simulink model "Task_f"  (R2025b)
settings: Solver=VariableStepAuto  StartTime=0.0  StopTime=10000  RelTol=1e-3
model workspace (MAT data in the model file):
  F = [0.06  0  0; 0  0.06  0; 0  0  0]
values from neighbouring files (symbols this model uses):
  A = [ -(1/(R1*C1) + 1/(R2*C1)),   1/(R2*C1),                 0 ... (first row only)    [Lab_Prep.m]    (also in Lab_Session.m = [ -(k1 + k12),      k12,            0)
  b = [1/(R1*C1); 0; 0]    [Lab_Prep.m]    (also in Lab_Session.m = [kin; 0; 0])
  C = [0, 0, 1]    [Lab_Prep.m]    (also in Lab_Session.m = [0 0 1])
  D = [0 0]    [Lab_Session.m]
settings Model: Creator=DemoBox  LastModifiedBy=DemoBox

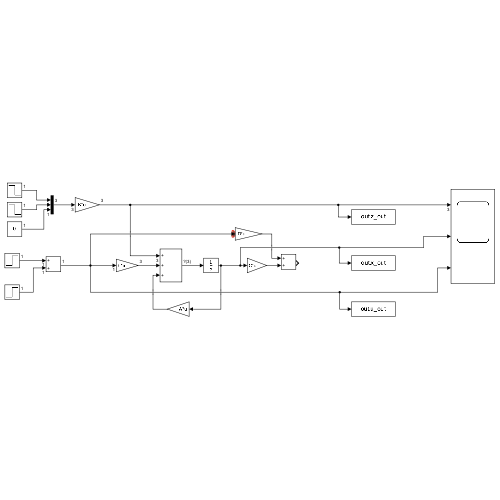
[thumbnail: Simulink's stored preview of the top-level diagram]
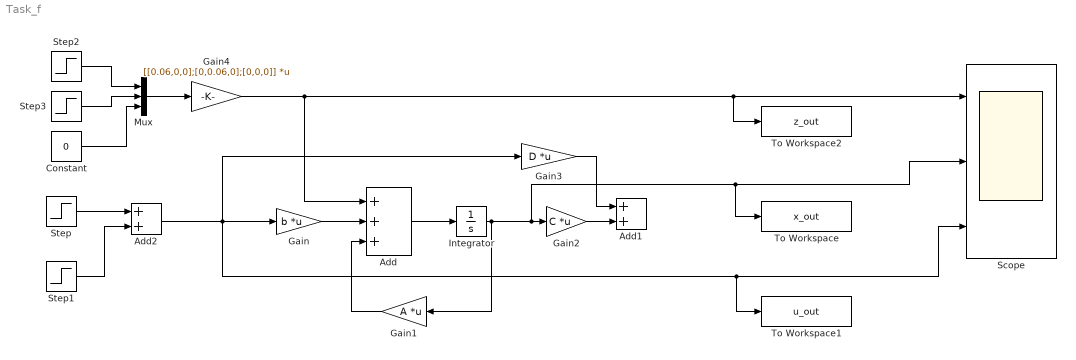
== system Task_f ==
  Add : Sum  Inputs=+++
  Add1 : Sum
  Add2 : Sum
  Constant : Constant  Value=0
  Gain : Gain  Gain=b  Multiplication=Matrix(K*u)
  Gain1 : Gain  Gain=A  Multiplication=Matrix(K*u)
  Gain2 : Gain  Gain=C  Multiplication=Matrix(K*u)
  Gain3 : Gain  Gain=D  Multiplication=Matrix(K*u)
  Gain4 : Gain  Gain=[[0.06,0,0];[0,0.06,0];[0,0,0]]  Multiplication=Matrix(K*u)
  Integrator : Integrator
  Mux : Mux  Inputs=3
  Scope : Scope  NumInputPorts=3
      settings: ActiveDisplayYMinimum=-26.584647265699061  ActiveDisplayYMaximum=74.463301350312619
  Step : Step  Time=0  After=0.1  SampleTime=0
  Step1 : Step  Time=2000  After=0.15  SampleTime=0
  Step2 : Step  Time=4000  After=-0.02  SampleTime=0
  Step3 : Step  Time=6000  After=-0.05  SampleTime=0
  To Workspace : ToWorkspace  VariableName=x_out  SaveFormat=Timeseries  SampleTime=-1
  To Workspace1 : ToWorkspace  VariableName=u_out  SaveFormat=Timeseries  SampleTime=-1
  To Workspace2 : ToWorkspace  VariableName=z_out  SaveFormat=Timeseries  SampleTime=-1
  wires:
  Gain1/1 -> Add/3
  Gain/1 -> Add/2
  Add/1 -> Integrator/1
  Integrator/1 -> Gain1/1, Scope/2, To Workspace/1, Gain2/1
  Gain2/1 -> Add1/2
  Gain3/1 -> Add1/1
  Mux/1 -> Gain4/1
  Step1/1 -> Add2/2
  Step/1 -> Add2/1
  Step2/1 -> Mux/1
  Step3/1 -> Mux/2
  Constant/1 -> Mux/3
  Gain4/1 -> Add/1, Scope/1, To Workspace2/1
  Add2/1 -> To Workspace1/1, Scope/3, Gain3/1, Gain/1
